simulink model "planta_misteriosa"  (R2018a)
settings: Solver=VariableStepAuto  StartTime=0.0  StopTime=20  RelTol=1e-9
values from neighbouring files (symbols this model uses):
  G_pol = iv4(z_id,[4 4 1])    [identificar_planta_misteriosa.m]
  Ts = 1    [ejemplo_identificacion_LS.m]    (also in ejemplo_pipeline_identificacion.m; identificacion_LC.m; identificar_planta_misteriosa.m = 0.1)
libraries: simulink x2
settings Model: Creator=pablo  LastModifiedBy=pablo
settings OptimizationCC: BlockReduction=off  DefaultParameterBehavior=Inlined  BufferReuse=off

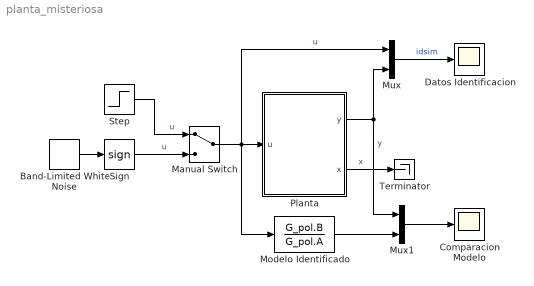
== system planta_misteriosa ==
  Band-Limited White Noise : simulink/Sources/Band-Limited White Noise  Cov=[0.1/3]  Ts=0.1  seed=[23341]
  Comparacion Modelo : Scope
  Datos Identificacion : Scope
  Manual Switch : ManualSwitch
  Modelo Identificado : DiscreteTransferFcn  Numerator=G_pol.B  Denominator=G_pol.A  SampleTime=Ts
  Mux : Mux  Inputs=2
  Mux1 : Mux  Inputs=2
  Planta : Subsystem
  Sign : Signum
  Step : Step  SampleTime=0
  Terminator : Terminator
  wires:
  Planta/1("y ") -> Mux1/1, Mux/2  "y"
  Mux/1 -> Datos Identificacion/1  "idsim"
  Band-Limited White Noise/1 -> Sign/1
  Manual Switch/1 -> Planta/1(u), Modelo Identificado/1, Mux/1  "u"
  Mux1/1 -> Comparacion Modelo/1
  Modelo Identificado/1 -> Mux1/2
  Step/1 -> Manual Switch/1  "u"
  Sign/1 -> Manual Switch/2  "u"
  Planta/2(x) -> Terminator/1  "x"

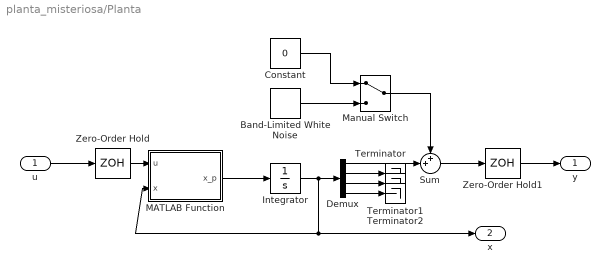
== system planta_misteriosa/Planta ==
  u : Inport
  Band-Limited White Noise : simulink/Sources/Band-Limited White Noise  Cov=[0.000001]  Ts=0.01  seed=[23341]
  Constant : Constant  Value=0
  Demux : Demux
  Integrator : Integrator  InitialCondition=[0 0 0 0]
  MATLAB Function : MATLAB Function  TreatAsAtomicUnit=on
  Manual Switch : ManualSwitch
  Sum : Sum  Inputs=++|
  Terminator : Terminator
  Terminator1 : Terminator
  Terminator2 : Terminator
  Zero-Order Hold : ZeroOrderHold  SampleTime=0.1
  Zero-Order Hold1 : ZeroOrderHold  SampleTime=0.1
  "y " : Outport
  x : Outport  Port=2
  wires:
  Zero-Order Hold1/1 -> "y "/1
  Zero-Order Hold/1 -> MATLAB Function/1(u)
  MATLAB Function/1(x_p) -> Integrator/1
  u/1 -> Zero-Order Hold/1
  Integrator/1 -> Demux/1, MATLAB Function/2(x), x/1
  Sum/1 -> Zero-Order Hold1/1
  Demux/1 -> Sum/2
  Band-Limited White Noise/1 -> Manual Switch/2
  Manual Switch/1 -> Sum/1
  Constant/1 -> Manual Switch/1
  Demux/2 -> Terminator/1
  Demux/3 -> Terminator1/1
  Demux/4 -> Terminator2/1

== matlab function planta_misteriosa/Planta/MATLAB Function ==
  data: u input; x_p output; x input
function x_p = fcn(u,x)

% recupero el estado
q = x(1);
qm = x(2);
q_p = x(3);
qm_p = x(4);

% El input es una tensión de +/- 10V
if u>10
    u=10;
elseif u<-10
    u=-10;
end
    
% El pendulo es una barra de ae m de largo y be x ce m de seccion
g = 9.8;
ae = 0.2;
be = 0.03;
ce = 0.01;
rho =  2700; %Kg/m3
m = rho*ae*be*ce;
xg = ae/2;
Igzz = m*(ae^2+be^2)/12;
Iozz = Igzz + m*xg^2;
b = 0.01*0;
Ke = 0.3;

N = 4; % Reducción
Jm = 0.395/(100*100); % kg m2
Bm = 0.05*0.6/(1000*2*pi)*60;
Km = 0.1*32/100/10; % Nm/Volt

tau_e = Ke*(qm-q);
qm_2p = (N*Km * u - Bm*N^2*qm_p - tau_e)/(Jm*N^2);
q_2p = (tau_e-m*g*xg*sin(q)-b*q_p)/Iozz;

x_p = [q_p; qm_p; q_2p; qm_2p];
